simulink model "power_3phseriescomp"  (Simulink 6.0)
settings: Solver=FixedStepDiscrete  StartTime=0.0  StopTime=0.2  FixedStep=Ts  RelTol=1e-4
InitFcn:
  | Ts=50e-6;
undefined symbols (not defined in the file or in its folder): D1, Delta, DiscIntNeverNeededParam
libraries: powerlib x54
settings Model: Creator=sybille  LastModifiedBy=batserve  ExtModeTrigMode=oneshot  ExtModeArmWhenConnect=off  ExtModeAutoUpdateStatusClock=off  ProdHWDeviceType=Specified
settings DataIOCC: LimitDataPoints=off  SignalLoggingName=sigsOut
settings OptimizationCC: BlockReduction=off  BooleanDataType=off
settings DebuggingCC: AlgebraicLoopMsg=none  CheckExecutionContextPreStartOutputMsg=on  CheckExecutionContextRuntimeOutputMsg=on  SolverPrmCheckMsg=none  UnconnectedInputMsg=none  UnconnectedOutputMsg=none
settings HardwareCC: ProdBitPerShort=32  ProdBitPerInt=16  ProdHWDeviceType=Specified  TargetUnknown=on

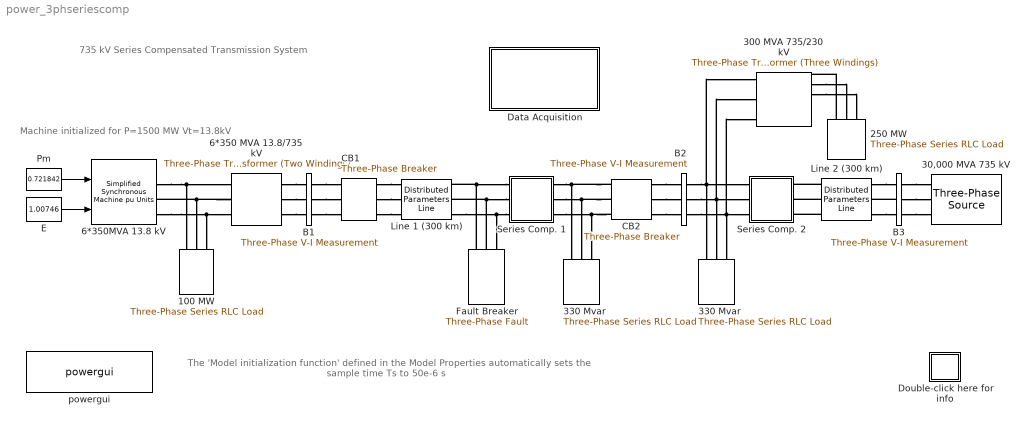
== system power_3phseriescomp ==
  note: Machine initialized for
      |  P=1500 MW
      |  Vt=13.8kV
  note: 735 kV Series Compensated Transmission System
  note: The 'Model  initialization function' defined in the
      | Model Properties automatically sets the sample time Ts
      | to 50e-6 s
  100 MW : powerlib/Elements/Three-Phase Series RLC Load  Orientation=down  PhysicalDomain=powersysdomain  SubClassName=unknown  LeftPortType=p1  RightPortType=p1  LConnTagsString=A|B|C  Configuration=Y (grounded)  NominalVoltage=13.8e3  NominalFrequency=60  ActivePower=100e6  InductivePower=0  CapacitivePower=0  Measurements=None
  250 MW : powerlib/Elements/Three-Phase Series RLC Load  Orientation=down  PhysicalDomain=powersysdomain  SubClassName=unknown  LeftPortType=p1  RightPortType=p1  LConnTagsString=A|B|C  Configuration=Y (grounded)  NominalVoltage=230e3  NominalFrequency=60  ActivePower=250e6  InductivePower=0  CapacitivePower=0  Measurements=None
  30,000 MVA 735 kV : powerlib/Electrical Sources/Three-Phase Source  Orientation=left  Voltage=735e3  PhaseAngle=0  Frequency=60  InternalConnection=Yg  SpecifyImpedance=on  Resistance=735^2/30000/10  Inductance=735^2/30000/377  ShortCircuitLevel=30000e6  BaseVoltage=735e3  XRratio=10
  300 MVA 735/230 kV : powerlib/Elements/Three-Phase Transformer (Three Windings)  NominalPower=[ 300e6 , 60 ]  Winding1Connection=Yg  Winding1=[ 735e3 , 0.002 , 0.15 ]  Winding2Connection=Yg  Winding2=[ 230e3 , 0.002 , 0 ]  Winding3Connection=Delta (D1)  Winding3=[ 25e3 , 0.05 , 0.20 ]  SetSaturation=on  Rm=500  Lm=1000  Saturation="[  0,0  ;  0.0012,1.2  ;  1.0,1.45 ]"  Hysteresis=off  DataFile='hysteresis'  SetInitialFlux=off  InitialFluxes=[-1.02651077007071 0.48004961184079 0.546461158229956]  Measurements=None  TransfoNumber=0
      settings: AttributesFormatString=\n
  330 Mvar : powerlib/Elements/Three-Phase Series RLC Load  Orientation=down  PhysicalDomain=powersysdomain  SubClassName=unknown  LeftPortType=p1  RightPortType=p1  LConnTagsString=A|B|C  Configuration=Y (grounded)  NominalVoltage=735e3  NominalFrequency=60  ActivePower=330e6/250  InductivePower=330e6  CapacitivePower=0  Measurements=None
  "330 Mvar " : powerlib/Elements/Three-Phase Series RLC Load  Orientation=down  PhysicalDomain=powersysdomain  SubClassName=unknown  LeftPortType=p1  RightPortType=p1  LConnTagsString=A|B|C  Configuration=Y (grounded)  NominalVoltage=735e3  NominalFrequency=60  ActivePower=330e6/250  InductivePower=330e6  CapacitivePower=0  Measurements=None
  6*350 MVA 13.8/735 kV : powerlib/Elements/Three-Phase Transformer (Two Windings)  NominalPower=[ 6*350e6 , 60 ]  Winding1Connection=Delta (D1)  Winding1=[ 13.8e3 , 0.002 , 0.08 ]  Winding2Connection=Yg  Winding2=[ 735e3 , 0.002 , 0.08 ]  SetSaturation=off  Rm=500  Lm=500  Saturation=[ 0,0 ; 0.0024,1.2 ; 1.0,1.52 ]  Hysteresis=off  DataFile='hysteresis'  SetInitialFlux=off  InitialFluxes=[ 0.8 , -0.8 , 0.7 ]  Measurements=None  TransfoNumber=0
  6*350MVA 13.8 kV : powerlib/Machines/Simplified Synchronous Machine pu Units  ConnectionType=3-wire Y  NominalParameters="[ 6*350e6 13.8e3  60 ]"  Mechanical=[ inf,0,2 ]  InternalRL="[ 0.22/15  0.22 ]"  InitialConditions=[0 3.29695 0.717757 0.717757 0.717757 -0.0992806 -120.099 119.901]  Units=0  LoadFlowParameters=[1,0,0,0,0]
      settings: AttributesFormatString=\n
  B1 : powerlib/Measurements/Three-Phase V-I Measurement  VoltageMeasurement=phase-to-ground  SetLabelV=on  LabelV=Vabc_B1  Vpu=on  Vbase=735e3  CurrentMeasurement=yes  SetLabelI=on  LabelI=Iabc_B1  Ipu=on  Pbase=100e6  OutputType=Complex  PhasorSimulation=off  PSBequivalent=0
  B2 : powerlib/Measurements/Three-Phase V-I Measurement  VoltageMeasurement=phase-to-ground  SetLabelV=on  LabelV=Vabc_B2  Vpu=on  Vbase=735e3  CurrentMeasurement=yes  SetLabelI=on  LabelI=Iabc_B2  Ipu=on  Pbase=100e6  OutputType=Complex  PhasorSimulation=off  PSBequivalent=0
  B3 : powerlib/Measurements/Three-Phase V-I Measurement  VoltageMeasurement=no  SetLabelV=on  LabelV=Vabc_B3  Vpu=on  Vbase=735e3  CurrentMeasurement=no  SetLabelI=on  LabelI=Iabc_B3  Ipu=on  Pbase=100e6  OutputType=Complex  PhasorSimulation=off  PSBequivalent=0
  CB1 : powerlib/Elements/Three-Phase Breaker  InitialState=closed  SwitchA=on  SwitchB=on  SwitchC=on  SwitchTimes="[5/60  ]"  External=off  BreakerResistance=0.001  SnubberResistance=1e5  SnubberCapacitance=inf  Measurements=None
      settings: AttributesFormatString=\n
  CB2 : powerlib/Elements/Three-Phase Breaker  InitialState=closed  SwitchA=on  SwitchB=on  SwitchC=on  SwitchTimes="[5/60  ]"  External=off  BreakerResistance=0.001  SnubberResistance=1e5  SnubberCapacitance=inf  Measurements=None
      settings: AttributesFormatString=\n
  Data Acquisition : Subsystem
      mask Type: Data Acquisition
      mask Display: disp('Open this block\nto visualize\nrecorded signals')
  Double-click here for info : Subsystem
      mask Display: disp('?')
  E : Constant  Value=1.00746
  Fault Breaker : powerlib/Elements/Three-Phase Fault  Orientation=down  FaultA=on  FaultB=off  FaultC=off  FaultResistance=0.001  GroundFault=on  GroundResistance=1  External=off  SwitchStatus=[1 0]  SwitchTimes=[ 1/60 6/60]  InitialStates=[0 0 1]  SnubberResistance=inf  SnubberCapacitance=inf  Measurements=Fault currents
  Line 1 (300 km) : powerlib/Elements/Distributed Parameters Line  Phases=3  Frequency=60  Resistance=[0.01273 0.3864]  Inductance="[0.9337e-3  4.1264e-3]"  Capacitance=[12.74e-9 7.751e-9]  Length=300  x1=[0 2.38552381946369e-008 325341.08168739 -670874.016355876;0.000339324940197445 1.66459232813684e-008 408268.627872248 -623887.123417706;0.000678649880394891 9.16458302355892e-009 484524.305378812 -566704.754576294;0.00101797482059234 1.53347643483349e-009 552861.954616155 -500261.376086399;0.00135729976078978 -6.12269001079985e-009 612164.811301234 -425642.796324084;0.00169662470098723 -1.36788003146648e-008 661463.756464234 -344068.421658456]  x2=[0 9.00972448785389e-009 143769.461527806 -735688.260633339;0.000339324940197445 6.80636344061194e-009 236449.298916992 -711335.722184491;0.000678649880394891 4.49177375626123e-009 325265.115012966 -675358.635091462;0.00101797482059234 2.10378013492283e-009 408765.494200877 -628344.931867615;0.00135729976078978 -3.18593166434968e-010 485585.884990611 -571062.903859812;0.00169662470098723 -2.73576006293297e-009 554470.899325939 -504448.64593894]  x3=[0 -3.13336489994457e-011 17.2118715948375 -960.069025644473;0.000339324940197445 -3.98990747122372e-011 139.55186503984 -950.027231912677;0.000678649880394891 -4.78124753398469e-011 259.611321471236 -924.460226348765;0.00101797482059234 -5.49445311986604e-011 375.428246084106 -883.785821373223;0.00135729976078978 -6.1178691231732e-011 485.109974933712 -828.668712409695;0.00169662470098723 -6.64130776698172e-011 586.86410458434 -760.009615525562]  x4=[0 1.02084477025663e-010 677.994740024314 -4520.13101941677;0.000339324940197445 1.00621023816259e-010 1249.10389719491 -4396.70345545888;0.000678649880394891 9.75132359425044e-011 1799.80037359926 -4201.42558004037;0.00101797482059234 9.28119004381258e-011 2321.08476462644 -3937.4885968238;0.00135729976078978 8.65938458688188e-011 2804.43831384126 -3609.20572698546;0.00169662470098723 7.89606868105969e-011 3241.96212530757 -3221.94172315972]  x5=0.00169662470098723  Measurements=None
      settings: AttributesFormatString=\n
  Line 2 (300 km) : powerlib/Elements/Distributed Parameters Line  Phases=3  Frequency=60  Resistance=[0.01273 0.3864]  Inductance="[0.9337e-3  4.1264e-3]"  Capacitance=[12.74e-9 7.751e-9]  Length=300  x1=[0 8.08804650517917e-009 273412.942916167 -687639.522621092;0.000339324940197445 5.25405198368107e-009 358903.648376035 -647140.343610795;0.000678649880394891 2.3341964812726e-009 438529.20073167 -596065.687832913;0.00101797482059234 -6.23804132783442e-010 510988.370369812 -535250.21015161;0.00135729976078978 -3.57161062715755e-009 575097.039698855 -465687.748576952;0.00169662470098723 -6.46105036139488e-009 629807.553832524 -388515.083103484]  x2=[0 3.75630740865473e-010 125044.833272501 -732127.227535099;0.000339324940197445 2.83265138171218e-010 217423.39752828 -710192.586932821;0.000678649880394891 1.8627045630214e-010 306248.85910395 -676652.07864238;0.00101797482059234 8.62317687508948e-011 390069.644759583 -632053.81694795;0.00135729976078978 -1.52161062757664e-011 467515.966967491 -577126.62038956;0.00169662470098723 -1.16415321826935e-010 537322.208787962 -512768.10151269]  x3=[0 -2.63936524665043e-011 22.3118706662993 -1296.73415864154;0.000339324940197445 -2.98432956179868e-011 187.559938160351 -1283.29090051926;0.000678649880394891 -3.28052438164469e-011 349.742927440492 -1248.87628241536;0.00101797482059234 -3.52310933196841e-011 506.210466833616 -1194.05270319403;0.00135729976078978 -3.70812012352156e-011 654.405585747377 -1119.71608210076;0.00169662470098723 -3.83253333588669e-011 791.906500325129 -1027.08121777562]  x4=[0 4.64670787248012e-011 405.125803062547 -4180.52806228976;0.000339324940197445 4.65573009140136e-011 935.140210240407 -4094.68646807245;0.000678649880394891 4.5886690218924e-011 1449.87268720719 -3941.93008166026;0.00101797482059234 4.44662056654932e-011 1940.91154798871 -3724.7552265038;0.00135729976078978 4.23190606131446e-011 2400.23230436467 -3446.71094363859;0.00169662470098723 3.94803434052984e-011 2820.32880093018 -3112.34099375399]  x5=0.00169662470098723  Measurements=None
      settings: AttributesFormatString=\n
  Pm : Constant  Value=0.721842
  Series Comp. 1 : Subsystem
      mask Display: plot(0,0,100,100,[25 45],[50 50], [45 45],[35 65],[55 55],[35 65], [55 75],[50 50])
  Series Comp. 2 : Subsystem
      mask Display: plot(0,0,100,100,[25 45],[50 50], [45 45],[35 65],[55 55],[35 65], [55 75],[50 50])
  powergui : powerlib/powergui  Priority=2  Frange=0:0.5:500  Ylog=off  Xlog=off  save=on  variable=Zmes  ZoomFFT=on  StartTime=0.0  cycles=1  DisplayStyle=off  fundamental=60  FreqAxis=off  MaxFrequency=1000  frequencyindice=1  frequencyindicesteady=1  RmsSteady=1  display=off  Ts=Ts  methode=off  frequency=60  echomessages=off
  wires:
  Pm/1 -> 6*350MVA 13.8 kV/1
  E/1 -> 6*350MVA 13.8 kV/2
  connections:
  6*350 MVA 13.8/735 kV/LConn2 -- 6*350MVA 13.8 kV/RConn2 -- 100 MW/LConn2
  6*350MVA 13.8 kV/RConn1 -- 6*350 MVA 13.8/735 kV/LConn1 -- 100 MW/LConn1
  6*350MVA 13.8 kV/RConn3 -- 6*350 MVA 13.8/735 kV/LConn3 -- 100 MW/LConn3
  6*350 MVA 13.8/735 kV/RConn2 -- B1/LConn2
  6*350 MVA 13.8/735 kV/RConn1 -- B1/LConn1
  6*350 MVA 13.8/735 kV/RConn3 -- B1/LConn3
  B1/RConn2 -- CB1/LConn2
  B1/RConn1 -- CB1/LConn1
  B1/RConn3 -- CB1/LConn3
  CB1/RConn2 -- Line 1 (300 km)/LConn2
  CB1/RConn1 -- Line 1 (300 km)/LConn1
  CB1/RConn3 -- Line 1 (300 km)/LConn3
  Fault Breaker/LConn2 -- Line 1 (300 km)/RConn2 -- Series Comp. 1/LConn2
  Fault Breaker/LConn1 -- Line 1 (300 km)/RConn1 -- Series Comp. 1/LConn1
  Line 1 (300 km)/RConn3 -- Fault Breaker/LConn3 -- Series Comp. 1/LConn3
  CB2/RConn2 -- B2/LConn2
  CB2/RConn1 -- B2/LConn1
  CB2/RConn3 -- B2/LConn3
  CB2/LConn2 -- 330 Mvar/LConn2 -- Series Comp. 1/RConn2
  CB2/LConn3 -- 330 Mvar/LConn3 -- Series Comp. 1/RConn3
  CB2/LConn1 -- 330 Mvar/LConn1 -- Series Comp. 1/RConn1
  B2/RConn2 -- "330 Mvar "/LConn2 -- 300 MVA 735/230 kV/LConn2 -- Series Comp. 2/LConn2
  B2/RConn3 -- "330 Mvar "/LConn3 -- 300 MVA 735/230 kV/LConn3 -- Series Comp. 2/LConn3
  B2/RConn1 -- "330 Mvar "/LConn1 -- 300 MVA 735/230 kV/LConn1 -- Series Comp. 2/LConn1
  300 MVA 735/230 kV/RConn2 -- 250 MW/LConn2
  250 MW/LConn1 -- 300 MVA 735/230 kV/RConn1
  300 MVA 735/230 kV/RConn3 -- 250 MW/LConn3
  Line 2 (300 km)/RConn1 -- B3/LConn1
  B3/LConn2 -- Line 2 (300 km)/RConn2
  Line 2 (300 km)/RConn3 -- B3/LConn3
  B3/RConn3 -- 30,000 MVA 735 kV/RConn3
  B3/RConn2 -- 30,000 MVA 735 kV/RConn2
  B3/RConn1 -- 30,000 MVA 735 kV/RConn1
  Line 2 (300 km)/LConn2 -- Series Comp. 2/RConn2
  Line 2 (300 km)/LConn1 -- Series Comp. 2/RConn1
  Line 2 (300 km)/LConn3 -- Series Comp. 2/RConn3

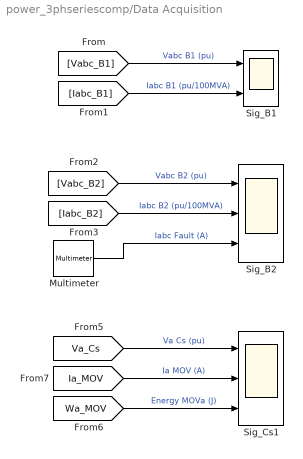
== system power_3phseriescomp/Data Acquisition ==
  Multimeter : powerlib/Measurements/Multimeter  Tag=PoWeRsYsTeMmEaSuReMeNt  PhasorSimulation=off  OutputType=Magnitude  sel=[1 2 3]  L=3  Gain=[1 1 1]  yselected={'Ib: Fault Breaker/Fault A','Ib: Fault Breaker/Fault B','Ib: Fault Breaker/Fault C'};  PSBOutputType=1  PSBequivalent=0  AxesSetting=[0,0.1,-100,100]  Display=0  SavedBlockNames={}
      settings: AttributesFormatString=\n
  Sig_B1 : Scope  NumInputPorts=2
      settings: TimeRange=0.2  YMin=-1.5~-20  YMax=1.5~40  SaveName=Sig_B1  SampleInput=on  SampleTime=Ts
  Sig_B2 : Scope  NumInputPorts=3
      settings: TimeRange=0.2  YMin=-2~-100~-10000  YMax=4~100~20000  SaveName=Sig_B2  SampleInput=on  SampleTime=Ts
  Sig_Cs1 : Scope  NumInputPorts=3
      settings: TimeRange=0.2  YMin=-300000~-10000~0  YMax=300000~15000~4e+007  SaveName=Sig_Cs1  SampleInput=on  SampleTime=Ts
  wires:
  [Vabc_B1] -> Sig_B1/1  "Vabc B1 (pu)"
  [Iabc_B1] -> Sig_B1/2  "Iabc B1 (pu/100MVA)"
  [Vabc_B2] -> Sig_B2/1  "Vabc B2 (pu)"
  [Iabc_B2] -> Sig_B2/2  "Iabc B2 (pu/100MVA)"
  [Va_Cs] -> Sig_Cs1/1  "Va Cs (pu)"
  [Ia_MOV] -> Sig_Cs1/2  "Ia MOV (A)"
  [Wa_MOV] -> Sig_Cs1/3  "Energy MOVa (J)"
  Multimeter/1 -> Sig_B2/3  "Iabc Fault (A)"

== system power_3phseriescomp/Double-click here for info ==
  note: G. Sybille (Hydro-Quebec)
  note: Demonstration
  note: This demonstration ilustrates use of  three-phase blocks
      | to study transients on a series-compensated 735-kV transmission system
  note: Circuit Description
  note: Fault and line switching:
  note: A three-phase, 60 Hz, 735 kV power system transmitting power from a power plant consisting of six 350 MVA generators to an equivalent network through a 600 km
      | transmission line. The transmission line is split in two 300 km lines connected between buses B1,B2, and B3. In order to increase the transmission capacity, each line
      | is series compensated by capacitors representing 40% of the line reactance. Both lines are also shunt compensated by a 330 Mvar shunt reactance. The shunt and series
      | compensation equipments are located at the B2 substation  where a 300 MVA 735/230 kV transformer with a 25 kV tertiary winding feeds a 230 kV, 250 MW load.
      | The series compensation subsystems are identical for the two lines. For each line Each phase containsof the series compensation module contains the series capacitor ,
      | a metal oxide varistor (MOV) protecting the capacitor, and a parallel gap protecting the MOV. When the energy dissipated in the MOV exceeds a threshold level of 30 MJ,
      | the gap simulated by a circuit breaker is fired. CB1 and CB2 are the the two line circuit breakers .
      |
      | The generators are simulated with a Simplified Synchronous Machine block. Universal transformer blocks (two-windings and three-windings) are used to model the two
      | transformers.  Saturation is implemented on the transformer connected at bus B2.  Voltages and currents are measured in B1, B2, and B3 blocks.
      | These blocks are Three-phase V-I Measurement blocks where  voltage and current  signals are sent to the Data Acquisition block through Goto blocks.
  note: You now study the transient performance of this circuit when a line-to-ground and three-phase-to-ground faults are applied on line 1.
      | The fault and the two line circuit breakers CB1 and CB2  are simulated with blocks from the three-phase library.
      | Open the dialog boxes of CB1 and CB2. See how the initial breaker status and switching times are specified.
      | A line-to-ground fault is applied on phase A at t = 1cycle. The two circuit breakers which are initially closed are then open at t = 5 cycles,
      | simulating a fault detection and opening time of 4 cycles. The fault is eliminated at t = 6 cycles, one cycle after line opening.
  note: Notice that this system contains the Powergui block. In addition, when you start the system the 'power_3phseriescomp' model, the  sampling time Ts = 50e-6 is
      | automatically set in your workspace. The system is therefore be discretized using a 50 microseconds sample time.
  note: Double click the Data Acquisition block and open the three scopes. Start the simulation.  As the system has already been initialized (1500 MW generation at the 13.8 kV bus)
      | with the Lod Flow utility of the Powergui, the simulation starts in steady state. At t = 1 cycle a line-to-ground fault is applied and the fault current reaches 10 kA .
      | During the fault, the MOV conducts at every half cycle and the energy dissipated in the MOV builds up to 13 MJ.
      |
      | At t = 5 cycles the line protection relays (not simulated) open breakers CB1 and CB2 and the energy stays constant at 13 MJ.  As the maximum energy does not exceed
      | the 30 MJ threshold level,  the gap is not fired. After breaker opening the fault current drops to a small value and the line and series capacitance start to discharge through the
      | fault and the shunt reactance. The fault current extinguishes at the first zero crossing after the opening order given to the fault breaker (t = 6 cycles). Then, the series capacitor
      | stops discharging and its voltage oscillates around 220 kV .
  note: Line-to-Ground Fault
  note: Three-Phase-to-Ground Fault
  note: Change the fault type to a three-phase-to-ground fault by checking Phases A, B, and C in in the Fault Breaker block.
      | Restart the simulation. Notice that during the fault the energy dissipated in the MOV builds up faster that in the case of a line-to-ground fault.
      | The energy reaches the 30 MJ threshold level after 3 cycles, one cycle before opening of the line breakers.
      | As a result, the gap is fired and the capacitor voltage quickly discharges to zero through the damping circuit.
  note: (See case study 'Series Compensated Transmission Network' in the SimPowerSystems User's Guide

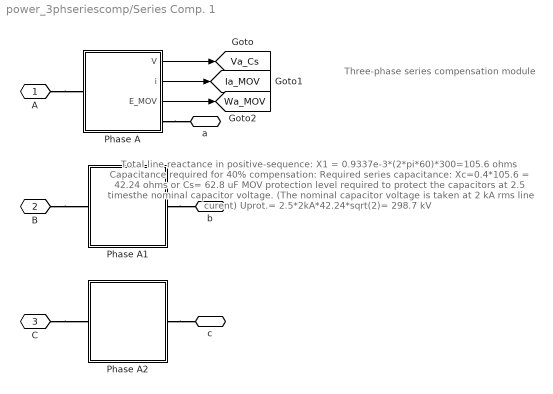
== system power_3phseriescomp/Series Comp. 1 ==
  note: Three-phase series compensation module
  note: Total line reactance in positive-sequence:
      |  X1 = 0.9337e-3*(2*pi*60)*300=105.6 ohms
      |
      | Capacitance required for 40% compensation:
      |
      | Required series capacitance:
      | Xc=0.4*105.6 = 42.24 ohms
      | or Cs= 62.8 uF
      |
      | MOV protection level required to protect the capacitors
      | at 2.5 timesthe nominal capacitor voltage.
      | (The nominal capacitor voltage is taken at 2 kA  rms line curent)
      |
      | Uprot.= 2.5*2kA*42.24*sqrt(2)= 298.7 kV
  Phase A : Subsystem
  Phase A1 : Subsystem
  Phase A2 : Subsystem
  A : PMIOPort  Port=1  Side=Left
  B : PMIOPort  Port=2  Side=Left
  C : PMIOPort  Port=3  Side=Left
  a : PMIOPort  Orientation=left  Port=4  Side=Right
  b : PMIOPort  Orientation=left  Port=5  Side=Right
  c : PMIOPort  Orientation=left  Port=6  Side=Right
  tag scope: Ia_MOV=global, Va_Cs=global, Wa_MOV=global
  wires:
  Phase A/2(i) -> [Ia_MOV]
  Phase A/1(V) -> [Va_Cs]
  Phase A/3(E_MOV) -> [Wa_MOV]
  connections:
  A/RConn1 -- Phase A/LConn1
  B/RConn1 -- Phase A1/LConn1
  C/RConn1 -- Phase A2/LConn1
  Phase A/RConn1 -- a/RConn1
  Phase A1/RConn1 -- b/RConn1
  Phase A2/RConn1 -- c/RConn1

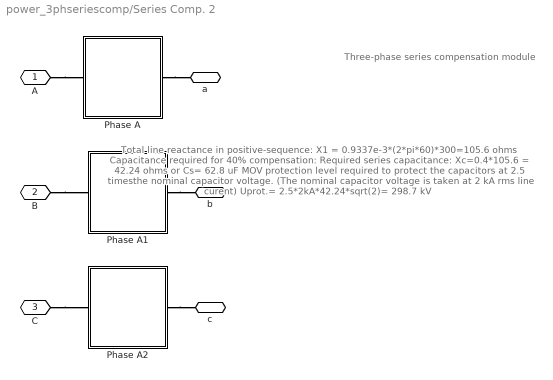
== system power_3phseriescomp/Series Comp. 2 ==
  note: Total line reactance in positive-sequence:
      |  X1 = 0.9337e-3*(2*pi*60)*300=105.6 ohms
      |
      | Capacitance required for 40% compensation:
      |
      | Required series capacitance:
      | Xc=0.4*105.6 = 42.24 ohms
      | or Cs= 62.8 uF
      |
      | MOV protection level required to protect the capacitors
      | at 2.5 timesthe nominal capacitor voltage.
      | (The nominal capacitor voltage is taken at 2 kA  rms line curent)
      |
      | Uprot.= 2.5*2kA*42.24*sqrt(2)= 298.7 kV
  note: Three-phase series compensation module
  Phase A : Subsystem
  Phase A1 : Subsystem
  Phase A2 : Subsystem
  A : PMIOPort  Port=1  Side=Left
  B : PMIOPort  Port=2  Side=Left
  C : PMIOPort  Port=3  Side=Left
  a : PMIOPort  Orientation=left  Port=4  Side=Right
  b : PMIOPort  Orientation=left  Port=5  Side=Right
  c : PMIOPort  Orientation=left  Port=6  Side=Right
  connections:
  Phase A2/RConn1 -- c/RConn1
  Phase A1/RConn1 -- b/RConn1
  Phase A/RConn1 -- a/RConn1
  C/RConn1 -- Phase A2/LConn1
  B/RConn1 -- Phase A1/LConn1
  A/RConn1 -- Phase A/LConn1

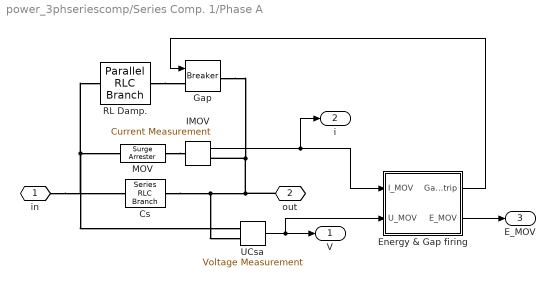
== system power_3phseriescomp/Series Comp. 1/Phase A ==
  Cs : powerlib/Elements/Series RLC Branch  PhysicalDomain=powersysdomain  SubClassName=unknown  LeftPortType=p1  RightPortType=p1  LConnTagsString=__new0  RConnTagsString=__new0  Resistance=0  Inductance=0  Capacitance=62.8e-6  Measurements=None
  Energy & Gap firing : Subsystem
  Gap : powerlib/Elements/Breaker  BreakerResistance=0.001  InitialState=0  SnubberResistance=inf  SnubberCapacitance=0  SwitchingTimes="[ 4/60  5/60 ]"  External=on  Measurements=None
      settings: AttributesFormatString=\n
  IMOV : powerlib/Measurements/Current Measurement  Tag=PoWeRsYsTeMmEaSuReMeNt  PhasorSimulation=off  OutputType=Magnitude  PSBequivalent=0
  MOV : powerlib/Elements/Surge Arrester  ProtectionVoltage=298.7e+03  Columns=60  ReferenceCurrent=500  Segment1=[.955 50]  Segment2=[1.0 25]  Segment3=[.9915 16.5]  Measurements=None  MoreParameters=off  BreakLoop=on
      settings: AttributesFormatString=\n
  RL Damp. : powerlib/Elements/Parallel RLC Branch  PhysicalDomain=powersysdomain  SubClassName=unknown  LeftPortType=p1  RightPortType=p1  LConnTagsString=a  RConnTagsString=__new0  Resistance=7.5  Inductance=1.7e-3  Capacitance=0  Measurements=None
  UCsa : powerlib/Measurements/Voltage Measurement  Tag=PoWeRsYsTeMmEaSuReMeNt  PhasorSimulation=off  OutputType=Magnitude  PSBequivalent=0
  in : PMIOPort  Port=1  Side=Left
  "out " : PMIOPort  Orientation=left  Port=2  Side=Right
  V : Outport
  i : Outport  Port=2
  E_MOV : Outport  Port=3
  wires:
  Energy & Gap firing/2(E_MOV) -> E_MOV/1
  IMOV/1 -> Energy & Gap firing/1(I_MOV), i/1
  UCsa/1 -> Energy & Gap firing/2(U_MOV), V/1
  Energy & Gap firing/1(Gap_trip) -> Gap/1
  connections:
  MOV/RConn1 -- IMOV/LConn1
  Cs/LConn1 -- UCsa/LConn1 -- in/RConn1 -- RL Damp./LConn1 -- MOV/LConn1
  RL Damp./RConn1 -- Gap/LConn1
  Cs/RConn1 -- "out "/RConn1 -- IMOV/RConn1 -- Gap/RConn1 -- UCsa/LConn2

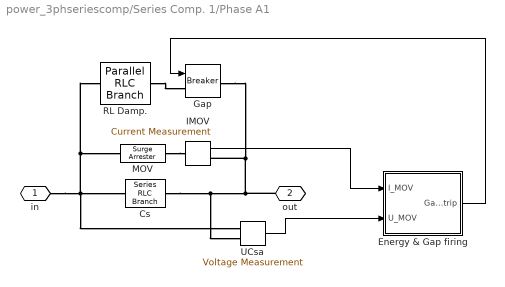
== system power_3phseriescomp/Series Comp. 1/Phase A1 ==
  Cs : powerlib/Elements/Series RLC Branch  PhysicalDomain=powersysdomain  SubClassName=unknown  LeftPortType=p1  RightPortType=p1  LConnTagsString=__new0  RConnTagsString=__new0  Resistance=0  Inductance=0  Capacitance=62.8e-6  Measurements=None
  Energy & Gap firing : Subsystem
  Gap : powerlib/Elements/Breaker  BreakerResistance=0.001  InitialState=0  SnubberResistance=inf  SnubberCapacitance=0  SwitchingTimes="[ 4/60  5/60 ]"  External=on  Measurements=None
      settings: AttributesFormatString=\n
  IMOV : powerlib/Measurements/Current Measurement  Tag=PoWeRsYsTeMmEaSuReMeNt  PhasorSimulation=off  OutputType=Magnitude  PSBequivalent=0
  MOV : powerlib/Elements/Surge Arrester  ProtectionVoltage=298.7e+03  Columns=60  ReferenceCurrent=500  Segment1=[.955 50]  Segment2=[1.0 25]  Segment3=[.9915 16.5]  Measurements=None  MoreParameters=off  BreakLoop=on
      settings: AttributesFormatString=\n
  RL Damp. : powerlib/Elements/Parallel RLC Branch  PhysicalDomain=powersysdomain  SubClassName=unknown  LeftPortType=p1  RightPortType=p1  LConnTagsString=a  RConnTagsString=__new0  Resistance=7.5  Inductance=1.7e-3  Capacitance=0  Measurements=None
  UCsa : powerlib/Measurements/Voltage Measurement  Tag=PoWeRsYsTeMmEaSuReMeNt  PhasorSimulation=off  OutputType=Magnitude  PSBequivalent=0
  in : PMIOPort  Port=1  Side=Left
  "out " : PMIOPort  Orientation=left  Port=2  Side=Right
  wires:
  Energy & Gap firing/1(Gap_trip) -> Gap/1
  UCsa/1 -> Energy & Gap firing/2(U_MOV)
  IMOV/1 -> Energy & Gap firing/1(I_MOV)
  connections:
  "out "/RConn1 -- UCsa/LConn2 -- Cs/RConn1 -- Gap/RConn1 -- IMOV/RConn1
  RL Damp./RConn1 -- Gap/LConn1
  in/RConn1 -- UCsa/LConn1 -- Cs/LConn1 -- MOV/LConn1 -- RL Damp./LConn1
  MOV/RConn1 -- IMOV/LConn1

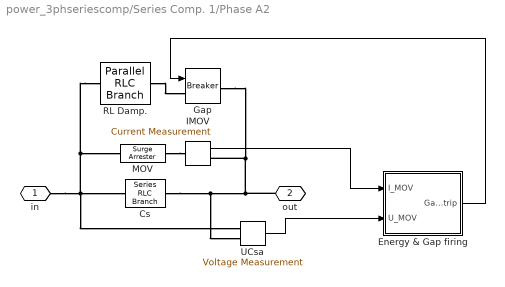
== system power_3phseriescomp/Series Comp. 1/Phase A2 ==
  Cs : powerlib/Elements/Series RLC Branch  PhysicalDomain=powersysdomain  SubClassName=unknown  LeftPortType=p1  RightPortType=p1  LConnTagsString=__new0  RConnTagsString=__new0  Resistance=0  Inductance=0  Capacitance=62.8e-6  Measurements=None
  Energy & Gap firing : Subsystem
  Gap : powerlib/Elements/Breaker  BreakerResistance=0.001  InitialState=0  SnubberResistance=inf  SnubberCapacitance=0  SwitchingTimes="[ 4/60  5/60 ]"  External=on  Measurements=None
      settings: AttributesFormatString=\n
  IMOV : powerlib/Measurements/Current Measurement  Tag=PoWeRsYsTeMmEaSuReMeNt  PhasorSimulation=off  OutputType=Magnitude  PSBequivalent=0
  MOV : powerlib/Elements/Surge Arrester  ProtectionVoltage=298.7e+03  Columns=60  ReferenceCurrent=500  Segment1=[.955 50]  Segment2=[1.0 25]  Segment3=[.9915 16.5]  Measurements=None  MoreParameters=off  BreakLoop=on
      settings: AttributesFormatString=\n
  RL Damp. : powerlib/Elements/Parallel RLC Branch  PhysicalDomain=powersysdomain  SubClassName=unknown  LeftPortType=p1  RightPortType=p1  LConnTagsString=a  RConnTagsString=__new0  Resistance=7.5  Inductance=1.7e-3  Capacitance=0  Measurements=None
  UCsa : powerlib/Measurements/Voltage Measurement  Tag=PoWeRsYsTeMmEaSuReMeNt  PhasorSimulation=off  OutputType=Magnitude  PSBequivalent=0
  in : PMIOPort  Port=1  Side=Left
  "out " : PMIOPort  Orientation=left  Port=2  Side=Right
  wires:
  IMOV/1 -> Energy & Gap firing/1(I_MOV)
  UCsa/1 -> Energy & Gap firing/2(U_MOV)
  Energy & Gap firing/1(Gap_trip) -> Gap/1
  connections:
  MOV/RConn1 -- IMOV/LConn1
  RL Damp./LConn1 -- MOV/LConn1 -- Cs/LConn1 -- UCsa/LConn1 -- in/RConn1
  RL Damp./RConn1 -- Gap/LConn1
  IMOV/RConn1 -- Gap/RConn1 -- Cs/RConn1 -- UCsa/LConn2 -- "out "/RConn1

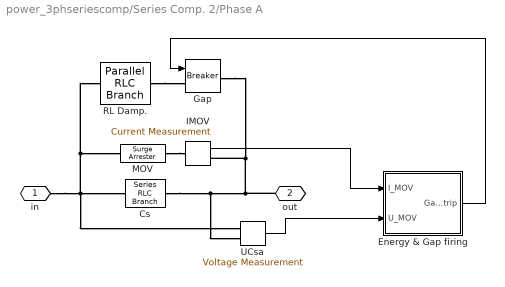
== system power_3phseriescomp/Series Comp. 2/Phase A ==
  Cs : powerlib/Elements/Series RLC Branch  PhysicalDomain=powersysdomain  SubClassName=unknown  LeftPortType=p1  RightPortType=p1  LConnTagsString=__new0  RConnTagsString=__new0  Resistance=0  Inductance=0  Capacitance=62.8e-6  Measurements=None
  Energy & Gap firing : Subsystem
  Gap : powerlib/Elements/Breaker  BreakerResistance=0.001  InitialState=0  SnubberResistance=inf  SnubberCapacitance=0  SwitchingTimes="[ 4/60  5/60 ]"  External=on  Measurements=None
      settings: AttributesFormatString=\n
  IMOV : powerlib/Measurements/Current Measurement  Tag=PoWeRsYsTeMmEaSuReMeNt  PhasorSimulation=off  OutputType=Magnitude  PSBequivalent=0
  MOV : powerlib/Elements/Surge Arrester  ProtectionVoltage=298.7e+03  Columns=60  ReferenceCurrent=500  Segment1=[.955 50]  Segment2=[1.0 25]  Segment3=[.9915 16.5]  Measurements=None  MoreParameters=off  BreakLoop=on
      settings: AttributesFormatString=\n
  RL Damp. : powerlib/Elements/Parallel RLC Branch  PhysicalDomain=powersysdomain  SubClassName=unknown  LeftPortType=p1  RightPortType=p1  LConnTagsString=a  RConnTagsString=__new0  Resistance=7.5  Inductance=1.7e-3  Capacitance=0  Measurements=None
  UCsa : powerlib/Measurements/Voltage Measurement  Tag=PoWeRsYsTeMmEaSuReMeNt  PhasorSimulation=off  OutputType=Magnitude  PSBequivalent=0
  in : PMIOPort  Port=1  Side=Left
  "out " : PMIOPort  Orientation=left  Port=2  Side=Right
  wires:
  Energy & Gap firing/1(Gap_trip) -> Gap/1
  UCsa/1 -> Energy & Gap firing/2(U_MOV)
  IMOV/1 -> Energy & Gap firing/1(I_MOV)
  connections:
  "out "/RConn1 -- UCsa/LConn2 -- Cs/RConn1 -- Gap/RConn1 -- IMOV/RConn1
  RL Damp./RConn1 -- Gap/LConn1
  in/RConn1 -- UCsa/LConn1 -- Cs/LConn1 -- MOV/LConn1 -- RL Damp./LConn1
  MOV/RConn1 -- IMOV/LConn1

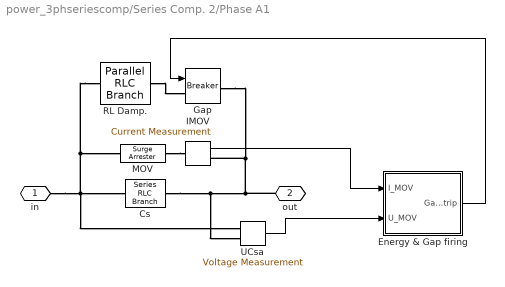
== system power_3phseriescomp/Series Comp. 2/Phase A1 ==
  Cs : powerlib/Elements/Series RLC Branch  PhysicalDomain=powersysdomain  SubClassName=unknown  LeftPortType=p1  RightPortType=p1  LConnTagsString=__new0  RConnTagsString=__new0  Resistance=0  Inductance=0  Capacitance=62.8e-6  Measurements=None
  Energy & Gap firing : Subsystem
  Gap : powerlib/Elements/Breaker  BreakerResistance=0.001  InitialState=0  SnubberResistance=inf  SnubberCapacitance=0  SwitchingTimes="[ 4/60  5/60 ]"  External=on  Measurements=None
      settings: AttributesFormatString=\n
  IMOV : powerlib/Measurements/Current Measurement  Tag=PoWeRsYsTeMmEaSuReMeNt  PhasorSimulation=off  OutputType=Magnitude  PSBequivalent=0
  MOV : powerlib/Elements/Surge Arrester  ProtectionVoltage=298.7e+03  Columns=60  ReferenceCurrent=500  Segment1=[.955 50]  Segment2=[1.0 25]  Segment3=[.9915 16.5]  Measurements=None  MoreParameters=off  BreakLoop=on
      settings: AttributesFormatString=\n
  RL Damp. : powerlib/Elements/Parallel RLC Branch  PhysicalDomain=powersysdomain  SubClassName=unknown  LeftPortType=p1  RightPortType=p1  LConnTagsString=a  RConnTagsString=__new0  Resistance=7.5  Inductance=1.7e-3  Capacitance=0  Measurements=None
  UCsa : powerlib/Measurements/Voltage Measurement  Tag=PoWeRsYsTeMmEaSuReMeNt  PhasorSimulation=off  OutputType=Magnitude  PSBequivalent=0
  in : PMIOPort  Port=1  Side=Left
  "out " : PMIOPort  Orientation=left  Port=2  Side=Right
  wires:
  IMOV/1 -> Energy & Gap firing/1(I_MOV)
  UCsa/1 -> Energy & Gap firing/2(U_MOV)
  Energy & Gap firing/1(Gap_trip) -> Gap/1
  connections:
  MOV/RConn1 -- IMOV/LConn1
  RL Damp./LConn1 -- MOV/LConn1 -- Cs/LConn1 -- UCsa/LConn1 -- in/RConn1
  RL Damp./RConn1 -- Gap/LConn1
  IMOV/RConn1 -- Gap/RConn1 -- Cs/RConn1 -- UCsa/LConn2 -- "out "/RConn1

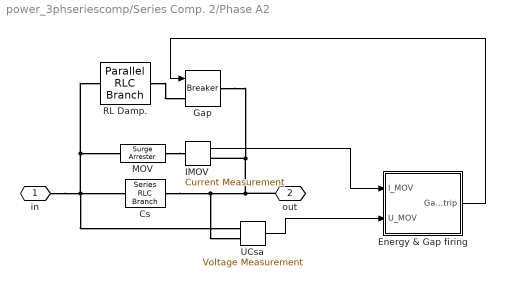
== system power_3phseriescomp/Series Comp. 2/Phase A2 ==
  Cs : powerlib/Elements/Series RLC Branch  PhysicalDomain=powersysdomain  SubClassName=unknown  LeftPortType=p1  RightPortType=p1  LConnTagsString=__new0  RConnTagsString=__new0  Resistance=0  Inductance=0  Capacitance=62.8e-6  Measurements=None
  Energy & Gap firing : Subsystem
  Gap : powerlib/Elements/Breaker  BreakerResistance=0.001  InitialState=0  SnubberResistance=inf  SnubberCapacitance=0  SwitchingTimes="[ 4/60  5/60 ]"  External=on  Measurements=None
      settings: AttributesFormatString=\n
  IMOV : powerlib/Measurements/Current Measurement  Tag=PoWeRsYsTeMmEaSuReMeNt  PhasorSimulation=off  OutputType=Magnitude  PSBequivalent=0
  MOV : powerlib/Elements/Surge Arrester  ProtectionVoltage=298.7e+03  Columns=60  ReferenceCurrent=500  Segment1=[.955 50]  Segment2=[1.0 25]  Segment3=[.9915 16.5]  Measurements=None  MoreParameters=off  BreakLoop=on
      settings: AttributesFormatString=\n
  RL Damp. : powerlib/Elements/Parallel RLC Branch  PhysicalDomain=powersysdomain  SubClassName=unknown  LeftPortType=p1  RightPortType=p1  LConnTagsString=a  RConnTagsString=__new0  Resistance=7.5  Inductance=1.7e-3  Capacitance=0  Measurements=None
  UCsa : powerlib/Measurements/Voltage Measurement  Tag=PoWeRsYsTeMmEaSuReMeNt  PhasorSimulation=off  OutputType=Magnitude  PSBequivalent=0
  in : PMIOPort  Port=1  Side=Left
  "out " : PMIOPort  Orientation=left  Port=2  Side=Right
  wires:
  Energy & Gap firing/1(Gap_trip) -> Gap/1
  UCsa/1 -> Energy & Gap firing/2(U_MOV)
  IMOV/1 -> Energy & Gap firing/1(I_MOV)
  connections:
  "out "/RConn1 -- UCsa/LConn2 -- Cs/RConn1 -- Gap/RConn1 -- IMOV/RConn1
  RL Damp./RConn1 -- Gap/LConn1
  in/RConn1 -- UCsa/LConn1 -- Cs/LConn1 -- MOV/LConn1 -- RL Damp./LConn1
  MOV/RConn1 -- IMOV/LConn1

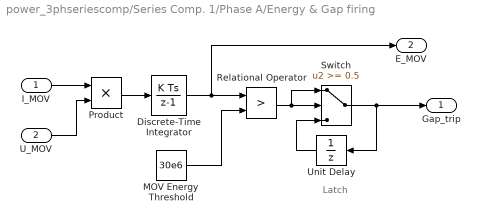
== system power_3phseriescomp/Series Comp. 1/Phase A/Energy & Gap firing ==
  note: Latch
  I_MOV : Inport  Port=1  LatchInput=off
  U_MOV : Inport  Port=2  LatchInput=off
  Discrete-Time Integrator : DiscreteIntegrator  SampleTime=Ts  ICPrevOutput=DiscIntNeverNeededParam  ICPrevScaledInput=DiscIntNeverNeededParam
  MOV Energy Threshold : Constant  Value=30e6
  Product : Product  SaturateOnIntegerOverflow=on  InputSameDT=on
  Relational Operator : RelationalOperator  Operator=>  ZeroCross=off  InputSameDT=on
  Switch : Switch  Threshold=0.5  ZeroCross=off  InputSameDT=on
  Unit Delay : UnitDelay  Orientation=left  SampleTime=Ts
  Gap_trip : Outport
  E_MOV : Outport  Port=2  InitialOutput=0
  wires:
  Switch/1 -> Unit Delay/1, Gap_trip/1
  U_MOV/1 -> Product/2
  MOV Energy Threshold/1 -> Relational Operator/2
  Product/1 -> Discrete-Time Integrator/1
  I_MOV/1 -> Product/1
  Discrete-Time Integrator/1 -> E_MOV/1, Relational Operator/1
  Relational Operator/1 -> Switch/1, Switch/2
  Unit Delay/1 -> Switch/3

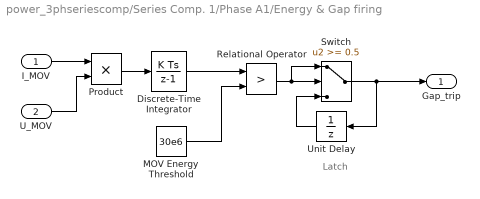
== system power_3phseriescomp/Series Comp. 1/Phase A1/Energy & Gap firing ==
  note: Latch
  I_MOV : Inport  Port=1  LatchInput=off
  U_MOV : Inport  Port=2  LatchInput=off
  Discrete-Time Integrator : DiscreteIntegrator  SampleTime=Ts  ICPrevOutput=DiscIntNeverNeededParam  ICPrevScaledInput=DiscIntNeverNeededParam
  MOV Energy Threshold : Constant  Value=30e6
  Product : Product  SaturateOnIntegerOverflow=on  InputSameDT=on
  Relational Operator : RelationalOperator  Operator=>  ZeroCross=off  InputSameDT=on
  Switch : Switch  Threshold=0.5  ZeroCross=off  InputSameDT=on
  Unit Delay : UnitDelay  Orientation=left  SampleTime=Ts
  Gap_trip : Outport
  wires:
  Unit Delay/1 -> Switch/3
  Relational Operator/1 -> Switch/2, Switch/1
  Discrete-Time Integrator/1 -> Relational Operator/1
  I_MOV/1 -> Product/1
  Product/1 -> Discrete-Time Integrator/1
  MOV Energy Threshold/1 -> Relational Operator/2
  U_MOV/1 -> Product/2
  Switch/1 -> Gap_trip/1, Unit Delay/1

== system power_3phseriescomp/Series Comp. 1/Phase A2/Energy & Gap firing ==
  note: Latch
  I_MOV : Inport  Port=1  LatchInput=off
  U_MOV : Inport  Port=2  LatchInput=off
  Discrete-Time Integrator : DiscreteIntegrator  SampleTime=Ts  ICPrevOutput=DiscIntNeverNeededParam  ICPrevScaledInput=DiscIntNeverNeededParam
  MOV Energy Threshold : Constant  Value=30e6
  Product : Product  SaturateOnIntegerOverflow=on  InputSameDT=on
  Relational Operator : RelationalOperator  Operator=>  ZeroCross=off  InputSameDT=on
  Switch : Switch  Threshold=0.5  ZeroCross=off  InputSameDT=on
  Unit Delay : UnitDelay  Orientation=left  SampleTime=Ts
  Gap_trip : Outport
  wires:
  Switch/1 -> Unit Delay/1, Gap_trip/1
  U_MOV/1 -> Product/2
  MOV Energy Threshold/1 -> Relational Operator/2
  Product/1 -> Discrete-Time Integrator/1
  I_MOV/1 -> Product/1
  Discrete-Time Integrator/1 -> Relational Operator/1
  Relational Operator/1 -> Switch/1, Switch/2
  Unit Delay/1 -> Switch/3

== system power_3phseriescomp/Series Comp. 2/Phase A/Energy & Gap firing ==
  note: Latch
  I_MOV : Inport  Port=1  LatchInput=off
  U_MOV : Inport  Port=2  LatchInput=off
  Discrete-Time Integrator : DiscreteIntegrator  SampleTime=Ts  ICPrevOutput=DiscIntNeverNeededParam  ICPrevScaledInput=DiscIntNeverNeededParam
  MOV Energy Threshold : Constant  Value=30e6
  Product : Product  SaturateOnIntegerOverflow=on  InputSameDT=on
  Relational Operator : RelationalOperator  Operator=>  ZeroCross=off  InputSameDT=on
  Switch : Switch  Threshold=0.5  ZeroCross=off  InputSameDT=on
  Unit Delay : UnitDelay  Orientation=left  SampleTime=Ts
  Gap_trip : Outport
  wires:
  Unit Delay/1 -> Switch/3
  Relational Operator/1 -> Switch/2, Switch/1
  Discrete-Time Integrator/1 -> Relational Operator/1
  I_MOV/1 -> Product/1
  Product/1 -> Discrete-Time Integrator/1
  MOV Energy Threshold/1 -> Relational Operator/2
  U_MOV/1 -> Product/2
  Switch/1 -> Gap_trip/1, Unit Delay/1

== system power_3phseriescomp/Series Comp. 2/Phase A1/Energy & Gap firing ==
  note: Latch
  I_MOV : Inport  Port=1  LatchInput=off
  U_MOV : Inport  Port=2  LatchInput=off
  Discrete-Time Integrator : DiscreteIntegrator  SampleTime=Ts  ICPrevOutput=DiscIntNeverNeededParam  ICPrevScaledInput=DiscIntNeverNeededParam
  MOV Energy Threshold : Constant  Value=30e6
  Product : Product  SaturateOnIntegerOverflow=on  InputSameDT=on
  Relational Operator : RelationalOperator  Operator=>  ZeroCross=off  InputSameDT=on
  Switch : Switch  Threshold=0.5  ZeroCross=off  InputSameDT=on
  Unit Delay : UnitDelay  Orientation=left  SampleTime=Ts
  Gap_trip : Outport
  wires:
  Switch/1 -> Unit Delay/1, Gap_trip/1
  U_MOV/1 -> Product/2
  MOV Energy Threshold/1 -> Relational Operator/2
  Product/1 -> Discrete-Time Integrator/1
  I_MOV/1 -> Product/1
  Discrete-Time Integrator/1 -> Relational Operator/1
  Relational Operator/1 -> Switch/1, Switch/2
  Unit Delay/1 -> Switch/3

== system power_3phseriescomp/Series Comp. 2/Phase A2/Energy & Gap firing ==
  note: Latch
  I_MOV : Inport  Port=1  LatchInput=off
  U_MOV : Inport  Port=2  LatchInput=off
  Discrete-Time Integrator : DiscreteIntegrator  SampleTime=Ts  ICPrevOutput=DiscIntNeverNeededParam  ICPrevScaledInput=DiscIntNeverNeededParam
  MOV Energy Threshold : Constant  Value=30e6
  Product : Product  SaturateOnIntegerOverflow=on  InputSameDT=on
  Relational Operator : RelationalOperator  Operator=>  ZeroCross=off  InputSameDT=on
  Switch : Switch  Threshold=0.5  ZeroCross=off  InputSameDT=on
  Unit Delay : UnitDelay  Orientation=left  SampleTime=Ts
  Gap_trip : Outport
  wires:
  Unit Delay/1 -> Switch/3
  Relational Operator/1 -> Switch/2, Switch/1
  Discrete-Time Integrator/1 -> Relational Operator/1
  I_MOV/1 -> Product/1
  Product/1 -> Discrete-Time Integrator/1
  MOV Energy Threshold/1 -> Relational Operator/2
  U_MOV/1 -> Product/2
  Switch/1 -> Gap_trip/1, Unit Delay/1
